simulink model "PID_Control_SystemFinalFinalll"  (R2024b)
settings: Solver=ode45  StartTime=0  StopTime=10  MaxStep=0.01  RelTol=1e-3
libraries: simulink_extras x1
settings Model: Creator=senac  LastModifiedBy=senac

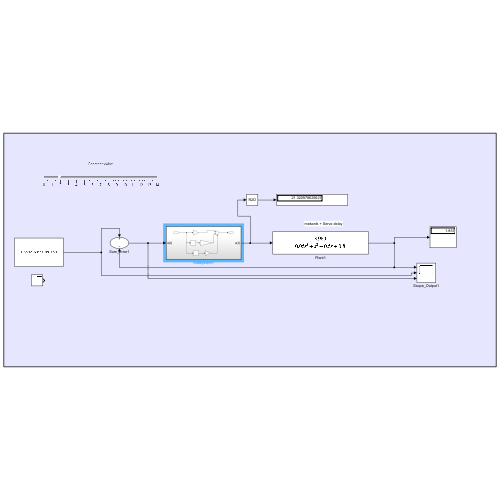
[thumbnail: Simulink's stored preview of the top-level diagram]
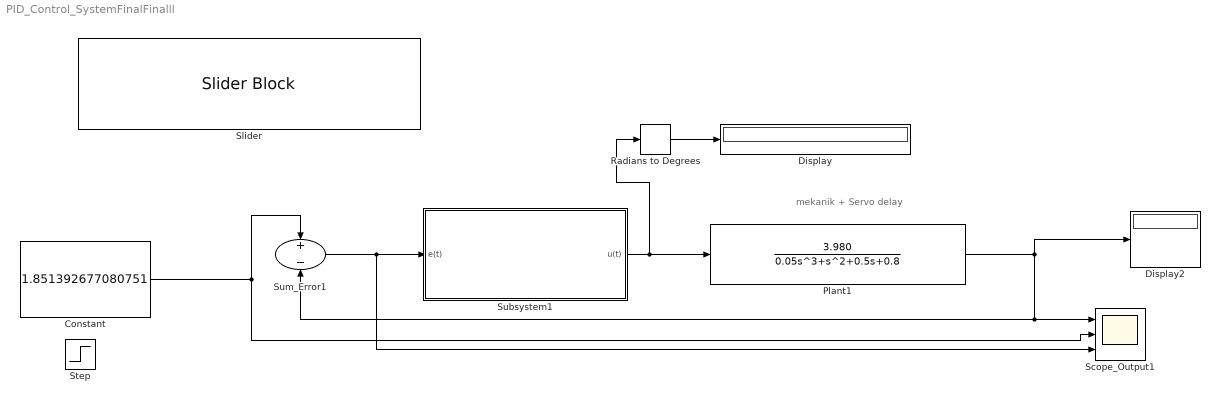
== system PID_Control_SystemFinalFinalll ==
  note: mekanik + Servo delay
  Constant : Constant  Value=1.851392677080751
  Display : Display
      settings: Format=decimal (Stored Integer)
  Display2 : Display
  Plant1 : TransferFcn  Numerator=[3.980]  Denominator="[0.05 1 0.5  0.8]"
  Radians to Degrees : simulink_extras/Transformations/Radians to Degrees
  Scope_Output1 : Scope  NumInputPorts=3
  Slider : SliderBlock  ScaleMax=14
  Step : Step  After=0.01  SampleTime=0
  Subsystem1 : Subsystem
  Sum_Error1 : Sum  Inputs=+-
  wires:
  Constant/1 -> Sum_Error1/1, Scope_Output1/2
  Plant1/1 -> Sum_Error1/2, Scope_Output1/1, Display2/1
  Sum_Error1/1 -> Scope_Output1/3, Subsystem1/1(e(t))
  Subsystem1/1(u(t)) -> Radians to Degrees/1, Plant1/1
  Radians to Degrees/1 -> Display/1

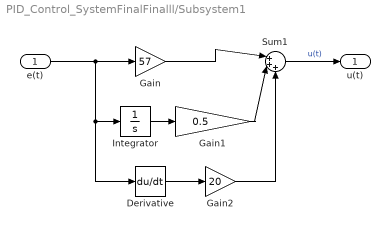
== system PID_Control_SystemFinalFinalll/Subsystem1 ==
  e(t) : Inport
  Derivative : Derivative
  Gain : Gain  Gain=57
  Gain1 : Gain  Gain=0.5
  Gain2 : Gain  Gain=20
  Integrator : Integrator
  Sum1 : Sum  Inputs=|+++
  u(t) : Outport
  wires:
  Sum1/1 -> u(t)/1  "u(t)"
  Gain2/1 -> Sum1/3
  e(t)/1 -> Gain/1, Derivative/1, Integrator/1
  Gain/1 -> Sum1/1
  Derivative/1 -> Gain2/1
  Gain1/1 -> Sum1/2
  Integrator/1 -> Gain1/1
